simulink model "parallel_two_level_spwm_2016"  (R2016a)
settings: Solver=VariableStepAuto  StartTime=0.0  StopTime=5  MaxStep=1e-4  RelTol=1e-3
libraries: powerlib x46, simulink x6, powerlib_meascontrol x3
settings Model: Creator=hakan  LastModifiedBy=hakan
settings DataIOCC: LimitDataPoints=on
settings DebuggingCC: MaxConsecutiveZCsMsg=none  AllowSymbolicDim=off
settings ModelReferenceCC: PropagateSignalLabelsOutOfModel=off
settings GRTTargetCC: GeneratePreprocessorConditionals=Use local settings

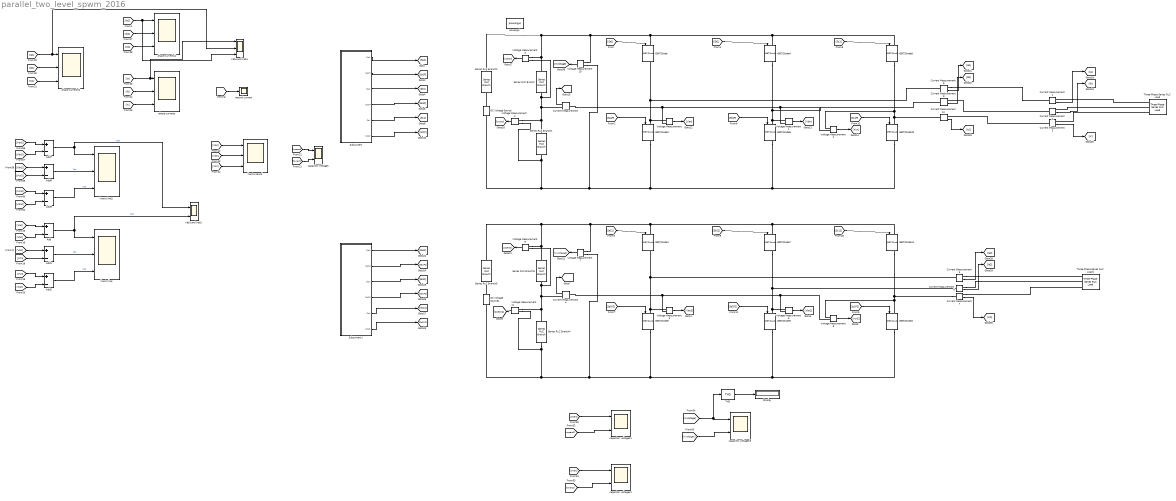
== system parallel_two_level_spwm_2016 ==
  Add{,1..2,7..9} (6 alike) : Sum  Inputs=+-
  Current Measurement{,1..10} (11 alike) : powerlib/Measurements/Current Measurement  PhasorSimulation=off  OutputType=Complex  PSBequivalent=0
  DC Voltage Source : powerlib/Electrical Sources/DC Voltage Source  Amplitude=540  Measurements=None
  DC Voltage Source1 : powerlib/Electrical Sources/DC Voltage Source  Amplitude=540  Measurements=None
  Display : Display
  IGBT/Diode{,1..11} (12 alike) : powerlib/Power Electronics/IGBT//Diode  Ron=1e-3  Rs=1e5  Cs=inf  Measurements=on
  Series RLC Branch{,1,3..4} (4 alike) : powerlib/Elements/Series RLC Branch  LConnTagsString=__new0  RConnTagsString=__new0  BranchType=C  Resistance=1  Inductance=1e-3  SetiL0=off  InitialCurrent=0  Capacitance=10e-6  Setx0=off  InitialVoltage=0  Measurements=None
  Series RLC Branch2 : powerlib/Elements/Series RLC Branch  LConnTagsString=__new0  RConnTagsString=__new0  BranchType=R  Resistance=1  Inductance=1e-3  SetiL0=off  InitialCurrent=0  Capacitance=1000e-6  Setx0=off  InitialVoltage=0  Measurements=None
  Series RLC Branch5 : powerlib/Elements/Series RLC Branch  LConnTagsString=__new0  RConnTagsString=__new0  BranchType=R  Resistance=1  Inductance=1e-3  SetiL0=off  InitialCurrent=0  Capacitance=1000e-6  Setx0=off  InitialVoltage=0  Measurements=None
  Subsystem : Subsystem
  Subsystem1 : Subsystem
  THD : powerlib_meascontrol/Measurements/THD  Freq=50  Ts=0
  Three-Phase Series RLC Load : powerlib/Elements/Three-Phase Series RLC Load  LConnTagsString=A|B|C  Configuration=Y (floating)  NominalVoltage=1000  Vabc=[1e3 1e3 1e3]  Vabcp=[1e3 1e3 1e3]  NominalFrequency=50  UnbalancedPower=off  ActivePower=8000  InductivePower=3870  CapacitivePower=0  Pabc=[10e3 9e3 11e3]  QLabc=[100 90 110]  QCabc=[100 90 110]  Pabcp=[10e3 9e3 11e3]  QLabcp=[100 90 110]  QCabcp=[100 90 110]  Measurements=None  LoadType=constant Z
  Three-Phase Series RLC Load1 : powerlib/Elements/Three-Phase Series RLC Load  LConnTagsString=A|B|C  Configuration=Y (floating)  NominalVoltage=1000  Vabc=[1e3 1e3 1e3]  Vabcp=[1e3 1e3 1e3]  NominalFrequency=50  UnbalancedPower=off  ActivePower=8000  InductivePower=3870  CapacitivePower=0  Pabc=[10e3 9e3 11e3]  QLabc=[100 90 110]  QCabc=[100 90 110]  Pabcp=[10e3 9e3 11e3]  QLabcp=[100 90 110]  QCabcp=[100 90 110]  Measurements=None  LoadType=constant Z
  Vab1 and Vab1 : Scope  NumInputPorts=3
  Vab1 and Vab2 : Scope  NumInputPorts=2
  Voltage Measurement{,1..11} (12 alike) : powerlib/Measurements/Voltage Measurement  PhasorSimulation=off  OutputType=Complex  PSBequivalent=0
  capacitor voltages{,1..3} (4 alike) : Scope  NumInputPorts=2
  line to line : Scope  NumInputPorts=3
  line to line2 : Scope  NumInputPorts=3
  line to neural : Scope  NumInputPorts=3
  neutral current : Scope
  phase currents : Scope  NumInputPorts=3
  phase currents1 : Scope  NumInputPorts=3
  phase currents2 : Scope  NumInputPorts=3
  powergui : powerlib/powergui  Priority=1  SimulationMode=Continuous  SolverType=Tustin/Backward Euler (TBE)  SampleTime=50e-6  frequency=60  SPID=on  DisableSnubberDevices=off  DisableRonSwitches=off  DisableVfSwitches=off  SwTol=0  DisplayEquations=off  Interpol=off  ExternalGateDelay=off  methode=off  Ts=100  FunctionMessages=off  echomessages=off  HookPort=off  EnableUseOfTLC=off  x0status=blocks  frequencyindice=0  Pbase=100e6  ErrMax=1e-4  Iterations=50  UnitsV=kV  UnitsW=MW  buscounter=0  RestoreLinks=warning  ResistiveCurrentMeasurement=off  Frange=[0:2:500]  Ylog=off  Xlog=on  ShowGrid=off  save=off  variable=ZData  structure=0  ZoomFFT=off  StartTime=0.0  cycles=1  DisplayStyle=1  fundamental=60  FreqAxis=off  MaxFrequency=1000  frequencyindicesteady=1  RmsSteady=1  display=off
  wires:
  Subsystem/1("Sa1 ") -> [Sa1]
  Subsystem/2(Sa1P) -> [Sa1P]
  Subsystem/3(Sb1) -> [Sb1]
  Subsystem/6(Sc1P) -> [Sc1P]
  Subsystem/5(Sc1) -> [Sc1]
  Subsystem/4(Sb1P) -> [Sb1P]
  [Sa1] -> IGBT/Diode/1
  [Sa1P] -> IGBT/Diode2/1
  [Sb1] -> IGBT/Diode4/1
  [Sb1P] -> IGBT/Diode6/1
  [Sc1] -> IGBT/Diode8/1
  [Sc1P] -> IGBT/Diode10/1
  Voltage Measurement/1 -> [Van]
  Voltage Measurement1/1 -> [Vbn]
  Voltage Measurement2/1 -> [Vcn]
  Voltage Measurement3/1 -> [upperc]
  Voltage Measurement4/1 -> [lowerc]
  Current Measurement/1 -> [Ineutral]
  [Ineutral] -> neutral current/1
  Current Measurement1/1 -> [Ia]
  Current Measurement2/1 -> [Ib]
  Current Measurement3/1 -> [Ic]
  [Ib] -> phase currents/2
  [Ia] -> Vab1 and Vab1/1, phase currents/1
  [Ic] -> phase currents/3
  [Van] -> Add/1
  [Vbn] -> Add/2
  [Vbn] -> Add1/1
  [Vcn] -> Add1/2
  Add1/1 -> line to line/2  "Vbc"
  [Vcn] -> Add2/1
  [Van] -> Add2/2
  Add2/1 -> line to line/3  "Vca"
  [Van] -> line to neural/1
  [Vbn] -> line to neural/2
  [Vcn] -> line to neural/3
  [lowerc] -> capacitor voltages/2
  [upperc] -> capacitor voltages/1
  Voltage Measurement10/1 -> [involtage]
  [Sa12] -> IGBT/Diode1/1
  [Sa1P2] -> IGBT/Diode5/1
  [Sb12] -> IGBT/Diode7/1
  [Sb1P2] -> IGBT/Diode9/1
  [Sc12] -> IGBT/Diode11/1
  [Sc1P2] -> IGBT/Diode3/1
  Voltage Measurement5/1 -> [Van2]
  Voltage Measurement6/1 -> [Vbn2]
  Voltage Measurement8/1 -> [Vcn2]
  Voltage Measurement9/1 -> [upperc2]
  Voltage Measurement11/1 -> [lowerc2]
  Current Measurement4/1 -> [Ineutral2]
  Voltage Measurement7/1 -> [involtage2]
  Subsystem1/1("Sa1 ") -> [Sa12]
  Subsystem1/2(Sa1P) -> [Sa1P2]
  Subsystem1/3(Sb1) -> [Sb12]
  Subsystem1/6(Sc1P) -> [Sc1P2]
  Subsystem1/5(Sc1) -> [Sc12]
  Subsystem1/4(Sb1P) -> [Sb1P2]
  Add/1 -> Vab1 and Vab2/2, line to line/1  "Vab"
  [Van2] -> Add7/1
  [Vbn2] -> Add7/2
  Add7/1 -> Vab1 and Vab2/1, line to line2/1  "Vab"
  [Vbn2] -> Add8/1
  [Vcn2] -> Add8/2
  Add8/1 -> line to line2/2  "Vbc"
  [Vcn2] -> Add9/1
  [Van2] -> Add9/2
  Add9/1 -> line to line2/3  "Vca"
  [upperc] -> capacitor voltages1/1
  [lowerc] -> capacitor voltages2/1
  [upperc2] -> capacitor voltages1/2
  [lowerc2] -> capacitor voltages2/2
  [involtage] -> THD/1, capacitor voltages3/1
  [involtage2] -> capacitor voltages3/2
  THD/1 -> Display/1
  Current Measurement7/1 -> [Ic2]
  Current Measurement6/1 -> [Ib2]
  Current Measurement5/1 -> [Ia2]
  [Ic2] -> phase currents1/3
  [Ia2] -> Vab1 and Vab1/3, phase currents1/1
  [Ib2] -> phase currents1/2
  Current Measurement8/1 -> [Ia1]
  Current Measurement9/1 -> [Ib1]
  Current Measurement10/1 -> [Ic1]
  [Ic1] -> phase currents2/3
  [Ia1] -> Vab1 and Vab1/2, phase currents2/1
  [Ib1] -> phase currents2/2
  connections:
  Voltage Measurement2/LConn2 -- Voltage Measurement1/LConn2 -- Voltage Measurement/LConn2 -- Current Measurement/LConn1
  Three-Phase Series RLC Load/LConn1 -- Current Measurement1/RConn1
  Three-Phase Series RLC Load/LConn3 -- Current Measurement3/RConn1
  Three-Phase Series RLC Load/LConn2 -- Current Measurement2/RConn1
  DC Voltage Source/RConn1 -- Series RLC Branch2/RConn1
  Voltage Measurement8/LConn2 -- Current Measurement4/LConn1 -- Voltage Measurement5/LConn2 -- Voltage Measurement6/LConn2
  DC Voltage Source1/RConn1 -- Series RLC Branch5/RConn1
  IGBT/Diode11/LConn1 -- IGBT/Diode7/LConn1 -- IGBT/Diode1/LConn1 -- Voltage Measurement7/LConn1 -- Series RLC Branch5/LConn1 -- Voltage Measurement9/LConn1 -- Series RLC Branch3/LConn1
  Series RLC Branch/RConn1 -- Voltage Measurement3/LConn2 -- Current Measurement/RConn1 -- Series RLC Branch1/LConn1 -- Voltage Measurement4/LConn1
  Voltage Measurement11/LConn2 -- Series RLC Branch4/RConn1 -- Voltage Measurement7/LConn2 -- IGBT/Diode9/RConn1 -- IGBT/Diode3/RConn1 -- IGBT/Diode5/RConn1 -- DC Voltage Source1/LConn1
  Voltage Measurement8/LConn1 -- Current Measurement7/LConn1 -- IGBT/Diode11/RConn1 -- IGBT/Diode3/LConn1
  Current Measurement2/LConn1 -- Current Measurement9/RConn1
  Current Measurement3/LConn1 -- Current Measurement10/RConn1
  IGBT/Diode4/RConn1 -- Current Measurement9/LConn1 -- Voltage Measurement1/LConn1 -- IGBT/Diode6/LConn1
  IGBT/Diode8/RConn1 -- Current Measurement10/LConn1 -- IGBT/Diode10/LConn1 -- Voltage Measurement2/LConn1
  Voltage Measurement/LConn1 -- Current Measurement8/LConn1 -- IGBT/Diode/RConn1 -- IGBT/Diode2/LConn1
  Current Measurement5/RConn1 -- Three-Phase Series RLC Load1/LConn1
  Voltage Measurement5/LConn1 -- Current Measurement5/LConn1 -- IGBT/Diode1/RConn1 -- IGBT/Diode5/LConn1
  Voltage Measurement6/LConn1 -- Current Measurement6/LConn1 -- IGBT/Diode7/RConn1 -- IGBT/Diode9/LConn1
  Current Measurement8/RConn1 -- Current Measurement1/LConn1
  Current Measurement6/RConn1 -- Three-Phase Series RLC Load1/LConn2
  Current Measurement7/RConn1 -- Three-Phase Series RLC Load1/LConn3
  Voltage Measurement9/LConn2 -- Series RLC Branch3/RConn1 -- Current Measurement4/RConn1 -- Voltage Measurement11/LConn1 -- Series RLC Branch4/LConn1
  Voltage Measurement10/LConn1 -- IGBT/Diode4/LConn1 -- IGBT/Diode8/LConn1 -- IGBT/Diode/LConn1 -- Series RLC Branch2/LConn1 -- Voltage Measurement3/LConn1 -- Series RLC Branch/LConn1
  IGBT/Diode2/RConn1 -- IGBT/Diode10/RConn1 -- IGBT/Diode6/RConn1 -- Voltage Measurement10/LConn2 -- Series RLC Branch1/RConn1 -- Voltage Measurement4/LConn2 -- DC Voltage Source/LConn1

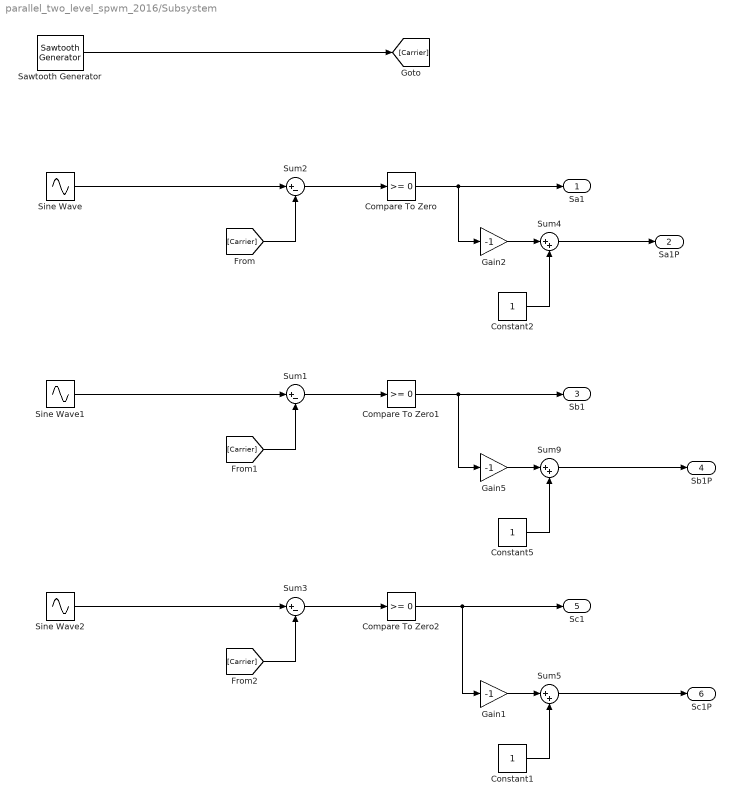
== system parallel_two_level_spwm_2016/Subsystem ==
  Compare To Zero : simulink/Logic and Bit Operations/Compare To Zero  relop=>=  OutDataTypeStr=boolean
  Compare To Zero1 : simulink/Logic and Bit Operations/Compare To Zero  relop=>=  OutDataTypeStr=boolean
  Compare To Zero2 : simulink/Logic and Bit Operations/Compare To Zero  relop=>=  OutDataTypeStr=boolean
  Constant1 : Constant
  Constant2 : Constant
  Constant5 : Constant
  Gain1 : Gain  Gain=-1
  Gain2 : Gain  Gain=-1
  Gain5 : Gain  Gain=-1
  Sawtooth Generator : powerlib_meascontrol/Pulse & Signal Generators/Sawtooth Generator  Freq=2050  Phase=0  Ts=0
  Sine Wave : Sin  Frequency=100*pi  SampleTime=0
  Sine Wave1 : Sin  Frequency=100*pi  Phase=2*pi/3  SampleTime=0
  Sine Wave2 : Sin  Frequency=100*pi  Phase=4*pi/3  SampleTime=0
  Sum1 : Sum  Inputs=|+-
  Sum2 : Sum  Inputs=|+-
  Sum3 : Sum  Inputs=|+-
  Sum4 : Sum  Inputs=|++
  Sum5 : Sum  Inputs=|++
  Sum9 : Sum  Inputs=|++
  "Sa1 " : Outport
  Sa1P : Outport  Port=2
  Sb1 : Outport  Port=3
  Sb1P : Outport  Port=4
  Sc1 : Outport  Port=5
  Sc1P : Outport  Port=6
  wires:
  Sine Wave/1 -> Sum2/1
  Sum4/1 -> Sa1P/1
  Gain2/1 -> Sum4/1
  Constant2/1 -> Sum4/2
  Compare To Zero/1 -> "Sa1 "/1, Gain2/1
  Sum2/1 -> Compare To Zero/1
  [Carrier] -> Sum2/2
  Sawtooth Generator/1 -> [Carrier]
  Compare To Zero1/1 -> Gain5/1, Sb1/1
  Sine Wave1/1 -> Sum1/1
  [Carrier] -> Sum1/2
  Compare To Zero2/1 -> Gain1/1, Sc1/1
  Sine Wave2/1 -> Sum3/1
  [Carrier] -> Sum3/2
  Sum1/1 -> Compare To Zero1/1
  Gain5/1 -> Sum9/1
  Sum9/1 -> Sb1P/1
  Constant5/1 -> Sum9/2
  Constant1/1 -> Sum5/2
  Sum5/1 -> Sc1P/1
  Sum3/1 -> Compare To Zero2/1
  Gain1/1 -> Sum5/1

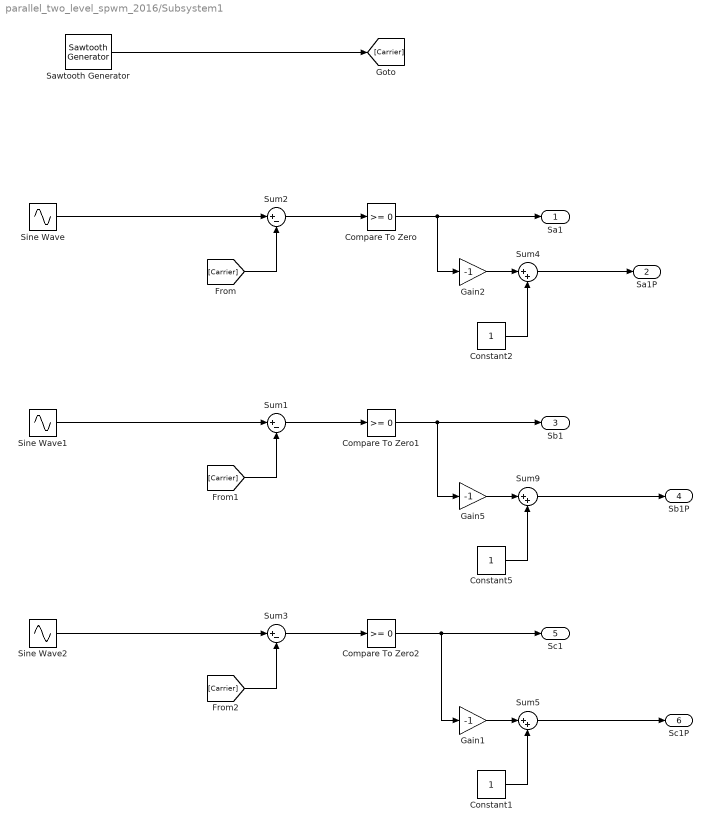
== system parallel_two_level_spwm_2016/Subsystem1 ==
  Compare To Zero : simulink/Logic and Bit Operations/Compare To Zero  relop=>=  OutDataTypeStr=boolean
  Compare To Zero1 : simulink/Logic and Bit Operations/Compare To Zero  relop=>=  OutDataTypeStr=boolean
  Compare To Zero2 : simulink/Logic and Bit Operations/Compare To Zero  relop=>=  OutDataTypeStr=boolean
  Constant1 : Constant
  Constant2 : Constant
  Constant5 : Constant
  Gain1 : Gain  Gain=-1
  Gain2 : Gain  Gain=-1
  Gain5 : Gain  Gain=-1
  Sawtooth Generator : powerlib_meascontrol/Pulse & Signal Generators/Sawtooth Generator  Freq=2050  Phase=180  Ts=0
  Sine Wave : Sin  Frequency=100*pi  SampleTime=0
  Sine Wave1 : Sin  Frequency=100*pi  Phase=2*pi/3  SampleTime=0
  Sine Wave2 : Sin  Frequency=100*pi  Phase=4*pi/3  SampleTime=0
  Sum1 : Sum  Inputs=|+-
  Sum2 : Sum  Inputs=|+-
  Sum3 : Sum  Inputs=|+-
  Sum4 : Sum  Inputs=|++
  Sum5 : Sum  Inputs=|++
  Sum9 : Sum  Inputs=|++
  "Sa1 " : Outport
  Sa1P : Outport  Port=2
  Sb1 : Outport  Port=3
  Sb1P : Outport  Port=4
  Sc1 : Outport  Port=5
  Sc1P : Outport  Port=6
  wires:
  Gain1/1 -> Sum5/1
  Sum3/1 -> Compare To Zero2/1
  Sum5/1 -> Sc1P/1
  Constant1/1 -> Sum5/2
  Constant5/1 -> Sum9/2
  Sum9/1 -> Sb1P/1
  Gain5/1 -> Sum9/1
  Sum1/1 -> Compare To Zero1/1
  [Carrier] -> Sum3/2
  Sine Wave2/1 -> Sum3/1
  Compare To Zero2/1 -> Sc1/1, Gain1/1
  [Carrier] -> Sum1/2
  Sine Wave1/1 -> Sum1/1
  Compare To Zero1/1 -> Sb1/1, Gain5/1
  Sawtooth Generator/1 -> [Carrier]
  [Carrier] -> Sum2/2
  Sum2/1 -> Compare To Zero/1
  Compare To Zero/1 -> Gain2/1, "Sa1 "/1
  Constant2/1 -> Sum4/2
  Gain2/1 -> Sum4/1
  Sum4/1 -> Sa1P/1
  Sine Wave/1 -> Sum2/1
